simulink model "seondrlc"  (R2022b)
settings: Solver=VariableStepAuto  StartTime=0.0  StopTime=0.55  RelTol=1e-3
libraries: simulink x1
settings Model: Creator=Asus  LastModifiedBy=Asus

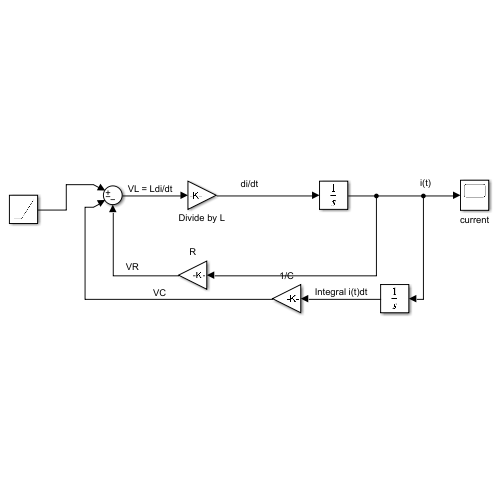
[thumbnail: Simulink's stored preview of the top-level diagram]
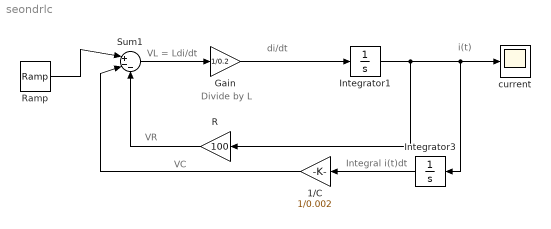
== system seondrlc ==
  note: VR
  note: Divide by L
  note: i(t)
  note: di/dt
  note: VC
  note: VL = Ldi/dt
  note: Integral i(t)dt
  1/C : Gain  Gain=1/0.002
  Gain : Gain  Gain=1/0.2
  Integrator1 : Integrator
  Integrator3 : Integrator
  R : Gain  Gain=100
  Ramp : simulink/Sources/Ramp  slope=1/5  start=0  InitialOutput=0
  Sum1 : Sum  Inputs=|+--
  current : Scope
  wires:
  Sum1/1 -> Gain/1
  Integrator1/1 -> R/1, Integrator3/1, current/1
  Gain/1 -> Integrator1/1
  R/1 -> Sum1/3
  Integrator3/1 -> 1/C/1
  1/C/1 -> Sum1/2
  Ramp/1 -> Sum1/1
